simulink model "Fsystem"  (R2020a)
settings: Solver=FixedStepAuto  StartTime=0.0  StopTime=20  FixedStep=1e-4  RelTol=1e-3
settings Model: Creator=hxk  LastModifiedBy=hxk

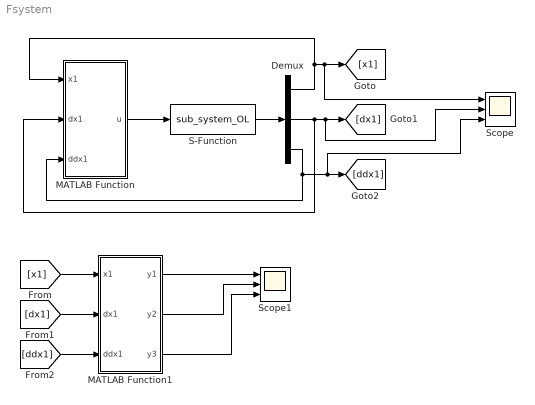
== system Fsystem ==
  Demux : Demux  Outputs=3
  MATLAB Function : MATLAB Function  TreatAsAtomicUnit=on
  MATLAB Function1 : MATLAB Function  TreatAsAtomicUnit=on
  S-Function : S-Function  FunctionName=sub_system_OL  SFunctionDeploymentMode=off  EnableBusSupport=off
  Scope : Scope  NumInputPorts=3
  Scope1 : Scope  NumInputPorts=3
  wires:
  MATLAB Function/1(u) -> S-Function/1
  S-Function/1 -> Demux/1
  Demux/1 -> Scope/1, [x1], MATLAB Function/1(x1)
  Demux/2 -> MATLAB Function/2(dx1), Scope/2, [dx1]
  Demux/3 -> Scope/3, [ddx1], MATLAB Function/3(ddx1)
  [x1] -> MATLAB Function1/1(x1)
  [dx1] -> MATLAB Function1/2(dx1)
  [ddx1] -> MATLAB Function1/3(ddx1)
  MATLAB Function1/1(y1) -> Scope1/1
  MATLAB Function1/2(y2) -> Scope1/2
  MATLAB Function1/3(y3) -> Scope1/3

== matlab function Fsystem/MATLAB Function1 ==
  data: x1 input; y1 output; dx1 input; ddx1 input; y2 output; y3 output
function [y1, y2, y3] = fcn(x1, dx1, ddx1)
g = x1-3.5; f = sin(x1); 
df = cos(x1)*dx1;
y1 = x1;
y2 = dx1-f;
y3 = (ddx1-df-x1*dx1+x1*f)/g;

== matlab function Fsystem/MATLAB Function ==
  data: x1 input; u output; dx1 input; ddx1 input
function u = fcn(x1, dx1, ddx1)
A = [6 11 6];
X = [x1;dx1;ddx1];
g = x1-3.5; f = sin(x1); 
dg = dx1; df = cos(x1)*dx1; ddf = -sin(x1)*dx1*dx1+cos(x1)*ddx1;
f1 = df+x1*(dx1-f);
df1 = ddf+dx1*(dx1-f)+x1*(ddx1-df);
f2 = g*df1+dg*(ddx1-f1);
u = -(A*X+f2/g)/g;
